simulink model "tf_rocketmodel_followref"  (R2019b)
settings: Solver=VariableStepAuto  StartTime=0.0  StopTime=60  RelTol=1e-3
values from neighbouring files (symbols this model uses):
  D = 0    [rocket_model.m]    (also in ss_model.mat; verif.m)
  g = 9.8    [main_rocketmodel.m]    (also in main_sim_rocket.m; rocket_model.m; sim_lin.m; test_bangbang.m)
  J_T = 40267    [main_rocketmodel.m]    (also in main_sim_rocket.m; rocket_model.m = 10)
  K_z = tf(lqg_ss)    [rocket_controllerdesign_z.m]
  m = 549054    [main_rocketmodel.m]    (also in main_sim_rocket.m; rocket_model.m = 25.4; sim_lin.m; test_bangbang.m)
  opt_controller = K_controller{k_min}    [main_yp_fminunc.m]    (also in reinforce_optim.m = s0_r0)
  s0_r0 = tf(sys_lqg)    [controller_design.m]    (also in main_sim_rocket.m = K_theta; main_yp_fminunc.m; sim_controller_design.m = tf(num{1},den{1}))
  sys = ss(A,B,C,D)    [controller_design.m]    (also in main_yp_fminunc.m; rocket_controllerdesign.m; rocket_controllerdesign_z.m; rocket_model.m)
  T = tf(8,[1,16,70,108,80])    [higher_order.m]    (also in rocket_model.m = 30; rocket_system.m = tf(omega^2, [1, 2*ksi*omega, omega^2]); second_order.m = tf(omega^2, [1, 2*ksi*omega, omega^2]))
  t_on = 14.6    [main_rocketmodel.m]    (also in main_sim_rocket.m; test_bangbang.m)
  Ts = 0.001    [main_rocketmodel.m]    (also in main_sim_rocket.m; sim_lin.m; square_sig.m; sum_squares_sig.m)
  Ts_sig = 0.001    [main_fmincon.m]    (also in main_reinforce.m; main_yp_fminunc.m; task1_disturb.m)
  x_0 = 0    [main_rocketmodel.m]    (also in main_sim_rocket.m)
  z_0 = 4000    [main_rocketmodel.m]    (also in main_sim_rocket.m; sim_lin.m; test_bangbang.m)
libraries: dspsrcs4 x1, simulink x1
settings Model: Creator=bia  LastModifiedBy=bia
settings DataIOCC: ExternalInput=[t,u,Fe]  LoadExternalInput=on

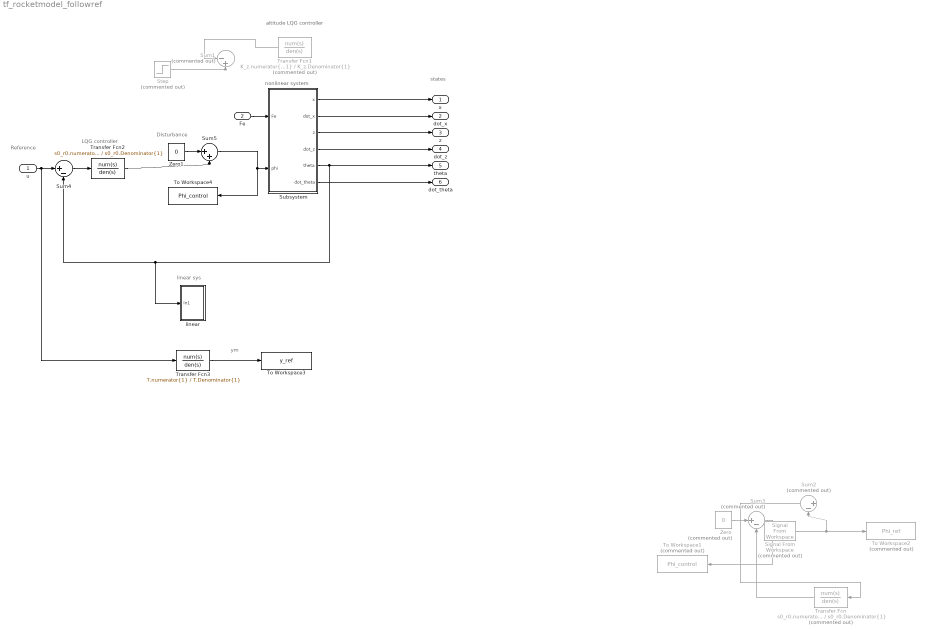
== system tf_rocketmodel_followref ==
  note: states
  note: altitude LQG controller
  note: nonlinear system
  note: LQG controller
  note: Reference
  note: Disturbance
  note: linear sys
  note: ym
  u : Inport
  Fe : Inport  Port=2
  Signal From Workspace : dspsrcs4/Signal From Workspace  Commented=on  X=ym  Ts=Ts_sig  nsamps=1  OutputAfterFinalValue=Setting to zero  ignoreOrWarnInputAndFrameLengths=off  OutputFrames=off
  Step : Step  Commented=on  Time=t_on  Before=0.05*7e6  After=7e6  SampleTime=0
  Subsystem : Subsystem
  Sum1 : Sum  Commented=on  Inputs=|-+
  Sum2 : Sum  Commented=on  Inputs=|+-
  Sum3 : Sum  Commented=on  Inputs=|+-
  Sum4 : Sum  Inputs=|+-
  Sum5 : Sum  Inputs=|++
  To Workspace1 : ToWorkspace  Commented=on  VariableName=Phi_control  SampleTime=Ts
  To Workspace2 : ToWorkspace  Commented=on  VariableName=Phi_ref  SampleTime=Ts
  To Workspace3 : ToWorkspace  VariableName=y_ref  SampleTime=Ts
  To Workspace4 : ToWorkspace  VariableName=Phi_control  SampleTime=Ts
  Transfer Fcn : TransferFcn  Commented=on  Numerator=s0_r0.numerator{1}  Denominator=s0_r0.Denominator{1}
  Transfer Fcn1 : TransferFcn  Commented=on  Numerator=K_z.numerator{1}  Denominator=K_z.Denominator{1}
  Transfer Fcn2 : TransferFcn  Numerator=s0_r0.numerator{1}  Denominator=s0_r0.Denominator{1}
  Transfer Fcn3 : TransferFcn  Numerator=T.numerator{1}  Denominator=T.Denominator{1}
  Zero : Constant  Commented=on  Value=0  OutDataTypeStr=Inherit: Inherit via back propagation  SampleTime=Ts
  Zero1 : Constant  Value=0  OutDataTypeStr=Inherit: Inherit via back propagation  SampleTime=Ts
  linear : Subsystem
  x : Outport
  "dot_x " : Outport  Port=2
  z : Outport  Port=3
  dot_z : Outport  Port=4
  theta : Outport  Port=5
  "dot_theta " : Outport  Port=6
  wires:
  Subsystem/6("dot_theta ") -> "dot_theta "/1
  Step/1 -> Sum1/2
  Subsystem/4("dot_z ") -> dot_z/1
  Subsystem/1(x) -> x/1
  Transfer Fcn1/1 -> Sum1/1
  Subsystem/3(z) -> z/1
  Subsystem/2(dot_x) -> "dot_x "/1
  Sum2/1 -> Transfer Fcn/1
  Signal From Workspace/1 -> Sum2/2, To Workspace2/1
  Transfer Fcn/1 -> Sum3/2
  Zero/1 -> Sum3/1
  Sum3/1 -> To Workspace1/1
  Sum4/1 -> Transfer Fcn2/1
  Transfer Fcn2/1 -> Sum5/2
  Subsystem/5(theta) -> theta/1, linear/1(In1), Sum4/2
  u/1 -> Transfer Fcn3/1, Sum4/1
  Zero1/1 -> Sum5/1
  Sum5/1 -> To Workspace4/1, Subsystem/2(phi)
  Fe/1 -> Subsystem/1(Fe)
  Transfer Fcn3/1 -> To Workspace3/1

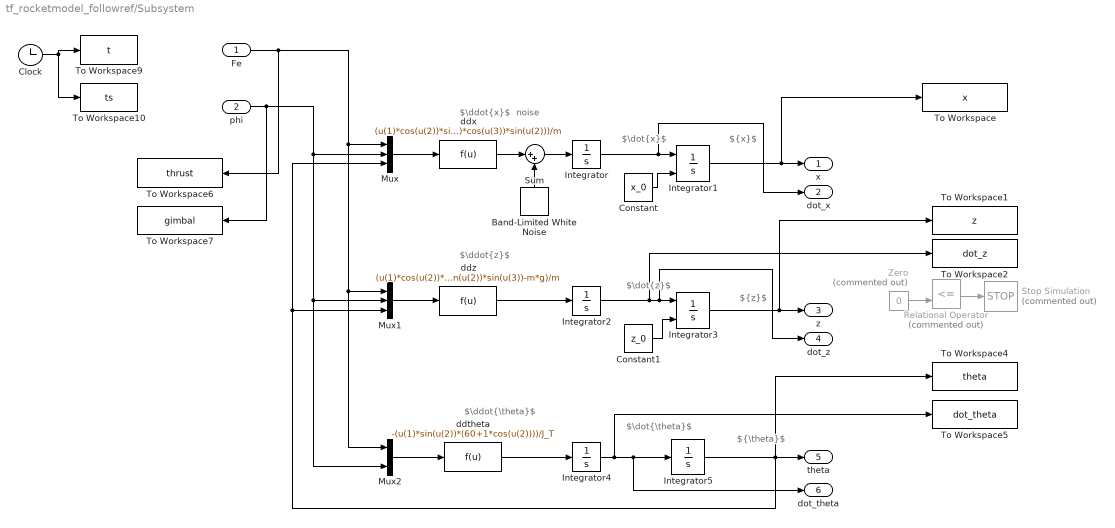
== system tf_rocketmodel_followref/Subsystem ==
  note: $\dot{z}$
  note: $\ddot{z}$
  note: ${z}$
  note: $\ddot{\theta}$
  note: $\ddot{x}$
  note: $\dot{x}$
  note: $\dot{\theta}$
  note: ${x}$
  note: ${\theta}$
  note: noise
  Fe : Inport
  phi : Inport  Port=2
  Band-Limited White Noise : simulink/Sources/Band-Limited White Noise  Cov=0  Ts=0.1  seed=[23341]
  Clock : Clock
  Constant : Constant  Value=x_0  SampleTime=Ts
  Constant1 : Constant  Value=z_0  SampleTime=Ts
  Integrator : Integrator  ContinuousStateAttributes='x_dot'
  Integrator1 : Integrator  InitialConditionSource=external  ContinuousStateAttributes='x'
  Integrator2 : Integrator  ContinuousStateAttributes='z_dot'
  Integrator3 : Integrator  InitialConditionSource=external  InitialCondition=50  LimitOutput=on  LowerSaturationLimit=0  ContinuousStateAttributes='z'
  Integrator4 : Integrator  ContinuousStateAttributes='theta_dot'
  Integrator5 : Integrator
  Mux : Mux  Inputs=3
  Mux1 : Mux  Inputs=3
  Mux2 : Mux  Inputs=2
  Relational Operator : RelationalOperator  Commented=on  Operator=<=  OutDataTypeStr=boolean  RndMeth=Nearest
  Stop Simulation : Stop  Commented=on
  Sum : Sum  Inputs=|++
  To Workspace : ToWorkspace  VariableName=x  SampleTime=Ts
  To Workspace1 : ToWorkspace  VariableName=z  SampleTime=Ts
  To Workspace10 : ToWorkspace  VariableName=ts  SampleTime=Ts
  To Workspace2 : ToWorkspace  VariableName=dot_z  SampleTime=Ts
  To Workspace4 : ToWorkspace  VariableName=theta  SampleTime=Ts
  To Workspace5 : ToWorkspace  VariableName=dot_theta  SampleTime=Ts
  To Workspace6 : ToWorkspace  VariableName=thrust  SampleTime=Ts
  To Workspace7 : ToWorkspace  VariableName=gimbal  SampleTime=Ts
  To Workspace9 : ToWorkspace  VariableName=t  SampleTime=-1
  Zero : Constant  Commented=on  Value=0  OutDataTypeStr=Inherit: Inherit via back propagation
  ddtheta : Fcn  Expr=-(u(1)*sin(u(2))*(60+1*cos(u(2))))/J_T
  ddx : Fcn  Expr=(u(1)*cos(u(2))*sin(u(3))+u(1)*cos(u(3))*sin(u(2)))/m
  ddz : Fcn  Expr=(u(1)*cos(u(2))*cos(u(3))-u(1)*sin(u(2))*sin(u(3))-m*g)/m
  x : Outport
  dot_x : Outport  Port=2
  z : Outport  Port=3
  "dot_z " : Outport  Port=4
  theta : Outport  Port=5
  "dot_theta " : Outport  Port=6
  wires:
  ddtheta/1 -> Integrator4/1
  Mux/1 -> ddx/1
  Integrator2/1 -> To Workspace2/1, "dot_z "/1, Integrator3/1
  Mux2/1 -> ddtheta/1
  Fe/1 -> To Workspace6/1, Mux2/1, Mux1/1, Mux/1
  Mux1/1 -> ddz/1
  Integrator/1 -> dot_x/1, Integrator1/1
  phi/1 -> To Workspace7/1, Mux2/2, Mux1/2, Mux/2
  Integrator3/1 -> z/1, To Workspace1/1
  Integrator5/1 -> To Workspace4/1, Mux1/3, Mux/3, theta/1
  Constant1/1 -> Integrator3/2
  Constant/1 -> Integrator1/2
  Integrator4/1 -> Integrator5/1, "dot_theta "/1, To Workspace5/1
  Zero/1 -> Relational Operator/2
  Relational Operator/1 -> Stop Simulation/1
  Clock/1 -> To Workspace9/1, To Workspace10/1
  ddz/1 -> Integrator2/1
  Integrator1/1 -> To Workspace/1, x/1
  Band-Limited White Noise/1 -> Sum/2
  Sum/1 -> Integrator/1
  ddx/1 -> Sum/1

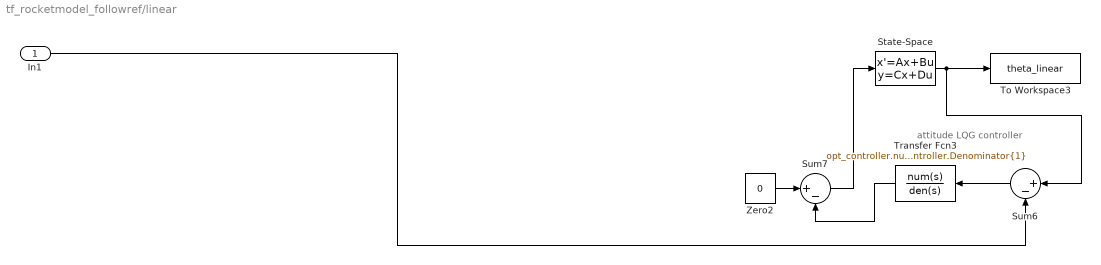
== system tf_rocketmodel_followref/linear ==
  note: attitude LQG controller
  In1 : Inport
  State-Space : StateSpace  A=sys.A  B=sys.B  C=sys.C  D=D  InitialCondition=0
  Sum6 : Sum  Inputs=|+-
  Sum7 : Sum  Inputs=|+-
  To Workspace3 : ToWorkspace  VariableName=theta_linear  SampleTime=Ts
  Transfer Fcn3 : TransferFcn  Numerator=opt_controller.numerator{1}  Denominator=opt_controller.Denominator{1}
  Zero2 : Constant  Value=0  OutDataTypeStr=Inherit: Inherit via back propagation  SampleTime=Ts
  wires:
  Transfer Fcn3/1 -> Sum7/2
  In1/1 -> Sum6/2
  Sum7/1 -> State-Space/1
  Sum6/1 -> Transfer Fcn3/1
  State-Space/1 -> To Workspace3/1, Sum6/1
  Zero2/1 -> Sum7/1
